simulink model "train_model_fessko2"  (R2021b)
settings: Solver=VariableStepAuto  StartTime=0.0  StopTime=15  RelTol=1e-3
model workspace (MAT data in the model file):
  b = 0.5
  g = 9.8
  l = 1
libraries: simulink_extras x1
settings Model: Creator=petr_  LastModifiedBy=petr_
settings DebuggingCC: UnconnectedInputMsg=none  UnconnectedOutputMsg=none  UnconnectedLineMsg=none
settings ModelReferenceCC: EnableRefExpFcnMdlSchedulingChecks=off
settings RTWCC: GPUComputeCapability=5.0  DLArmComputeVersion=20.02.1

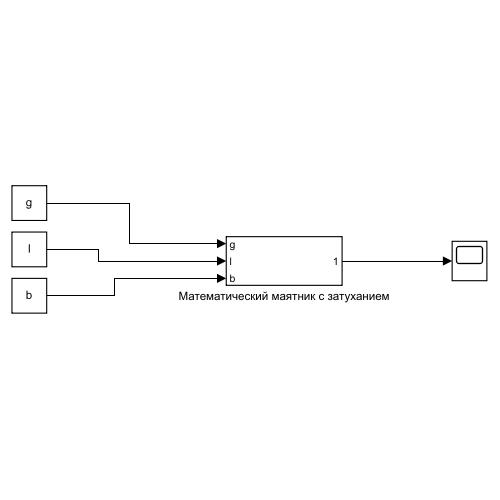
[thumbnail: Simulink's stored preview of the top-level diagram]
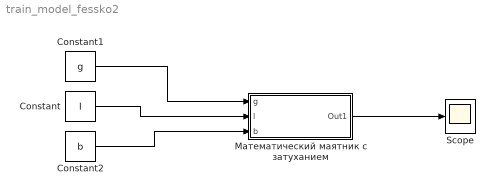
== system train_model_fessko2 ==
  Constant : Constant  Value=l  OutDataTypeStr=double
  Constant1 : Constant  Value=g  OutDataTypeStr=double
  Constant2 : Constant  Value=b  OutDataTypeStr=double
  Scope : Scope
  Математический маятник с затуханием : Subsystem
  wires:
  Математический маятник с затуханием/1(Out1) -> Scope/1
  Constant/1 -> Математический маятник с затуханием/2(l)
  Constant1/1 -> Математический маятник с затуханием/1(g)
  Constant2/1 -> Математический маятник с затуханием/3(b)

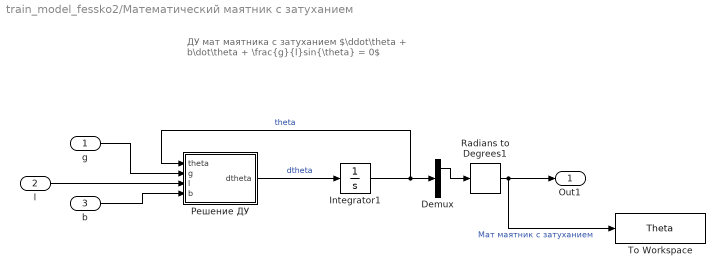
== system train_model_fessko2/Математический маятник с затуханием ==
  note: ДУ мат маятника с затуханием
      | $\ddot\theta + b\dot\theta + \frac{g}{l}sin{\theta} = 0$
  g : Inport
  l : Inport  Port=2
  b : Inport  Port=3
  Demux : Demux  Outputs=2
  Integrator1 : Integrator  InitialCondition=[deg2rad(30), 0]
  Radians to Degrees1 : simulink_extras/Transformations/Radians to Degrees
  To Workspace : ToWorkspace  VariableName=Theta  SaveFormat=Timeseries  SampleTime=-1
  Решение ДУ : MATLAB Function  TreatAsAtomicUnit=on
  Out1 : Outport
  wires:
  Integrator1/1 -> Решение ДУ/1(theta), Demux/1  "theta"
  Radians to Degrees1/1 -> To Workspace/1, Out1/1  "Мат маятник с затуханием"
  Решение ДУ/1(dtheta) -> Integrator1/1  "dtheta"
  g/1 -> Решение ДУ/2(g)
  l/1 -> Решение ДУ/3(l)
  b/1 -> Решение ДУ/4(b)
  Demux/1 -> Radians to Degrees1/1

== matlab function train_model_fessko2/Математический маятник с затуханием/Решение ДУ ==
  data: theta input; g input; dtheta output; l input; b input
function dtheta = fcn(theta, g, l, b)
dtheta = [theta(2), -g/l*sin(theta(1))-b*theta(2)];
